simulink model "lvbo"  (R2023a)
settings: Solver=VariableStepAuto  StartTime=0.0  StopTime=10000  RelTol=1e-3
libraries: dspfdesign x12
settings Model: Creator=wty  LastModifiedBy=wty

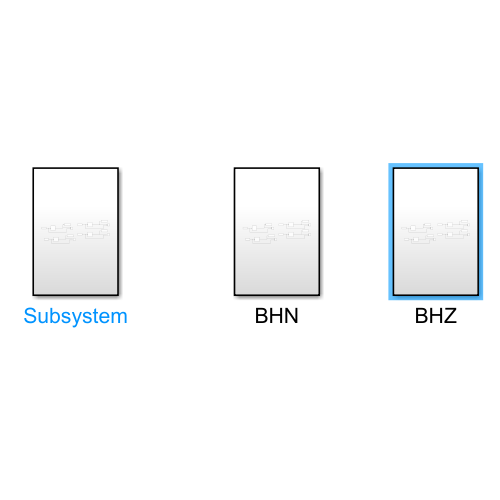
[thumbnail: Simulink's stored preview of the top-level diagram]
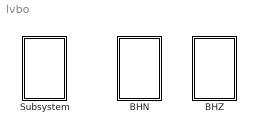
== system lvbo ==
  BHN : Subsystem
  BHZ : Subsystem
  Subsystem : Subsystem

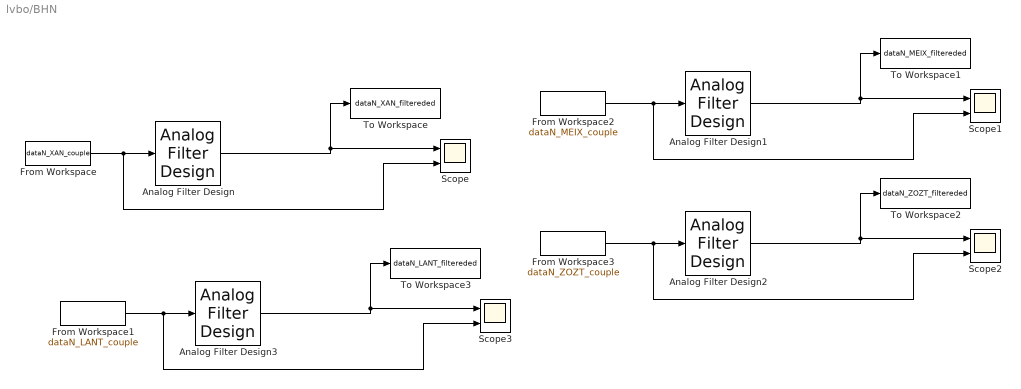
== system lvbo/BHN ==
  Analog Filter Design{,1..3} (4 alike) : dspfdesign/Analog Filter Design  method=Butterworth  filttype=Highpass  N=4  Wlo=0.0075  Whi=80  Rp=2  Rs=40
  From Workspace : FromWorkspace  VariableName=dataN_XAN_couple  OutputAfterFinalValue=Holding final value
  From Workspace1 : FromWorkspace  VariableName=dataN_LANT_couple  OutputAfterFinalValue=Holding final value
  From Workspace2 : FromWorkspace  VariableName=dataN_MEIX_couple  OutputAfterFinalValue=Holding final value
  From Workspace3 : FromWorkspace  VariableName=dataN_ZOZT_couple  OutputAfterFinalValue=Holding final value
  Scope{,1..3} (4 alike) : Scope  NumInputPorts=2
  To Workspace : ToWorkspace  VariableName=dataN_XAN_filtereded  SampleTime=-1
  To Workspace1 : ToWorkspace  VariableName=dataN_MEIX_filtereded  SampleTime=-1
  To Workspace2 : ToWorkspace  VariableName=dataN_ZOZT_filtereded  SampleTime=-1
  To Workspace3 : ToWorkspace  VariableName=dataN_LANT_filtereded  SampleTime=-1
  wires:
  Analog Filter Design/1 -> To Workspace/1, Scope/1
  Analog Filter Design1/1 -> To Workspace1/1, Scope1/1
  From Workspace2/1 -> Analog Filter Design1/1, Scope1/2
  Analog Filter Design3/1 -> To Workspace3/1, Scope3/1
  From Workspace1/1 -> Analog Filter Design3/1, Scope3/2
  From Workspace/1 -> Analog Filter Design/1, Scope/2
  From Workspace3/1 -> Analog Filter Design2/1, Scope2/2
  Analog Filter Design2/1 -> To Workspace2/1, Scope2/1

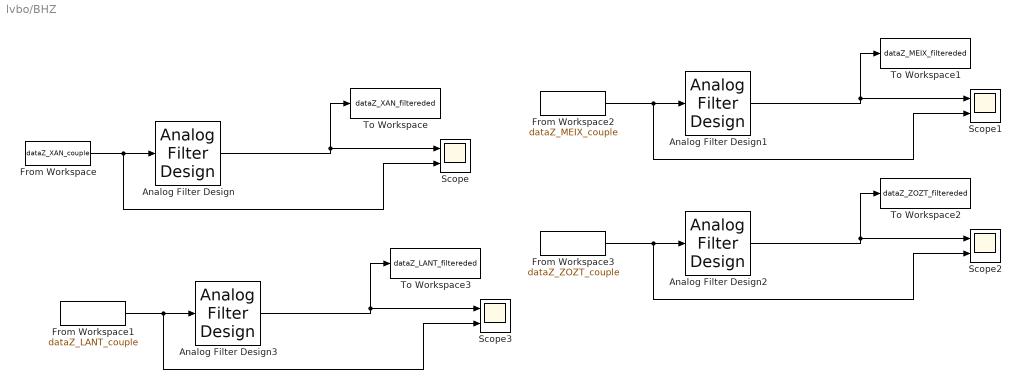
== system lvbo/BHZ ==
  Analog Filter Design{,1..3} (4 alike) : dspfdesign/Analog Filter Design  method=Butterworth  filttype=Highpass  N=4  Wlo=0.0075  Whi=80  Rp=2  Rs=40
  From Workspace : FromWorkspace  VariableName=dataZ_XAN_couple  OutputAfterFinalValue=Holding final value
  From Workspace1 : FromWorkspace  VariableName=dataZ_LANT_couple  OutputAfterFinalValue=Holding final value
  From Workspace2 : FromWorkspace  VariableName=dataZ_MEIX_couple  OutputAfterFinalValue=Holding final value
  From Workspace3 : FromWorkspace  VariableName=dataZ_ZOZT_couple  OutputAfterFinalValue=Holding final value
  Scope{,1..3} (4 alike) : Scope  NumInputPorts=2
  To Workspace : ToWorkspace  VariableName=dataZ_XAN_filtereded  SampleTime=-1
  To Workspace1 : ToWorkspace  VariableName=dataZ_MEIX_filtereded  SampleTime=-1
  To Workspace2 : ToWorkspace  VariableName=dataZ_ZOZT_filtereded  SampleTime=-1
  To Workspace3 : ToWorkspace  VariableName=dataZ_LANT_filtereded  SampleTime=-1
  wires:
  Analog Filter Design/1 -> To Workspace/1, Scope/1
  Analog Filter Design1/1 -> To Workspace1/1, Scope1/1
  From Workspace2/1 -> Analog Filter Design1/1, Scope1/2
  Analog Filter Design3/1 -> To Workspace3/1, Scope3/1
  From Workspace1/1 -> Analog Filter Design3/1, Scope3/2
  From Workspace/1 -> Analog Filter Design/1, Scope/2
  From Workspace3/1 -> Analog Filter Design2/1, Scope2/2
  Analog Filter Design2/1 -> To Workspace2/1, Scope2/1

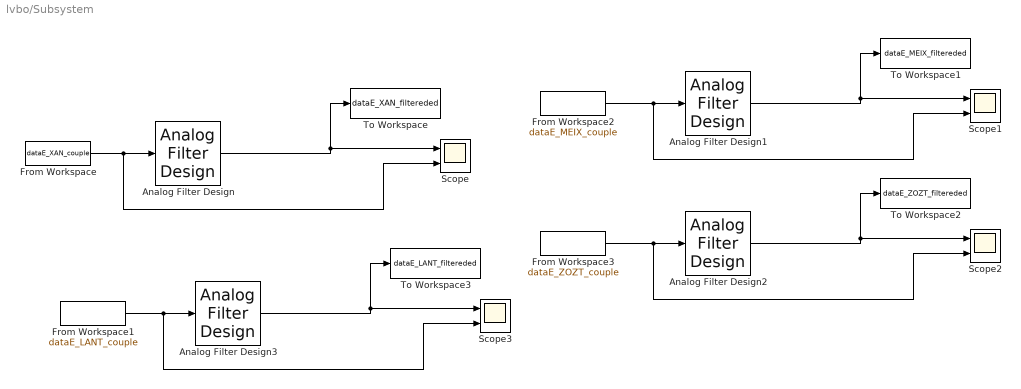
== system lvbo/Subsystem ==
  Analog Filter Design{,1..3} (4 alike) : dspfdesign/Analog Filter Design  method=Butterworth  filttype=Highpass  N=4  Wlo=0.0075  Whi=80  Rp=2  Rs=40
  From Workspace : FromWorkspace  VariableName=dataE_XAN_couple  OutputAfterFinalValue=Holding final value
  From Workspace1 : FromWorkspace  VariableName=dataE_LANT_couple  OutputAfterFinalValue=Holding final value
  From Workspace2 : FromWorkspace  VariableName=dataE_MEIX_couple  OutputAfterFinalValue=Holding final value
  From Workspace3 : FromWorkspace  VariableName=dataE_ZOZT_couple  OutputAfterFinalValue=Holding final value
  Scope{,1..3} (4 alike) : Scope  NumInputPorts=2
  To Workspace : ToWorkspace  VariableName=dataE_XAN_filtereded  SampleTime=-1
  To Workspace1 : ToWorkspace  VariableName=dataE_MEIX_filtereded  SampleTime=-1
  To Workspace2 : ToWorkspace  VariableName=dataE_ZOZT_filtereded  SampleTime=-1
  To Workspace3 : ToWorkspace  VariableName=dataE_LANT_filtereded  SampleTime=-1
  wires:
  Analog Filter Design/1 -> To Workspace/1, Scope/1
  Analog Filter Design1/1 -> To Workspace1/1, Scope1/1
  From Workspace2/1 -> Analog Filter Design1/1, Scope1/2
  Analog Filter Design3/1 -> To Workspace3/1, Scope3/1
  From Workspace1/1 -> Analog Filter Design3/1, Scope3/2
  From Workspace/1 -> Analog Filter Design/1, Scope/2
  From Workspace3/1 -> Analog Filter Design2/1, Scope2/2
  Analog Filter Design2/1 -> To Workspace2/1, Scope2/1
